simulink model "PMSM_vector_control_single"  (R2019a)
settings: Solver=ode4  StartTime=0.0  StopTime=Tfinal  FixedStep=Ts  RelTol=1e-3  EnableMultiTasking=on
values from neighbouring files (symbols this model uses):
  Cdc = 150e-6    (= 0.00015)    [PMSM_modular_vector_control_sim_parameters.m]    (also in PMSM_vector_control_single_parameters.m)
  IdPIDmax = Vdcm/5    (= 20)    [PMSM_modular_vector_control_sim_parameters.m]    (also in PMSM_vector_control_single_parameters.m)
  IdPIDmin = -Vdcm/5    (= -20)    [PMSM_modular_vector_control_sim_parameters.m]    (also in PMSM_vector_control_single_parameters.m)
  Idref = 0    [PMSM_vector_control_single_parameters.m]
  Inertia = 1e-2    (= 0.01)    [PMSM_modular_vector_control_sim_parameters.m]    (also in PMSM_vector_control_single_parameters.m)
  IqPIDmax = Vdcm-10    (= 90)    [PMSM_modular_vector_control_sim_parameters.m]    (also in PMSM_vector_control_single_parameters.m)
  IqPIDmin = -(Vdcm-10)    (= -90)    [PMSM_modular_vector_control_sim_parameters.m]    (also in PMSM_vector_control_single_parameters.m)
  IrefOverTref = MotorSpeedRad/(EfRated*3)    (= 0.261799387799)    [PMSM_modular_vector_control_sim_parameters.m]    (also in PMSM_vector_control_single_parameters.m)
  LoadTorque1 = 2    [PMSM_modular_vector_control_sim_parameters.m]    (also in PMSM_vector_control_single_parameters.m = 5)
  LoadTorque2 = 2    [PMSM_modular_vector_control_sim_parameters.m]    (also in PMSM_vector_control_single_parameters.m = 5)
  LoadTorqueStepTime = 3    [PMSM_modular_vector_control_sim_parameters.m]    (also in PMSM_vector_control_single_parameters.m)
  phase = [0 0 0 0]    [PMSM_modular_vector_control_sim_parameters.m]    (also in PMSM_vector_control_single_parameters.m)
  PolePairs = 10    [PMSM_modular_vector_control_sim_parameters.m]    (also in PMSM_vector_control_single_parameters.m)
  Rin = 1e-3    (= 0.001)    [PMSM_modular_vector_control_sim_parameters.m]    (also in PMSM_vector_control_single_parameters.m)
  Rs = 321e-3    (= 0.321)    [PMSM_modular_vector_control_sim_parameters.m]    (also in PMSM_vector_control_single_parameters.m)
  SpeedPIDmax = 20    [PMSM_modular_vector_control_sim_parameters.m]    (also in PMSM_vector_control_single_parameters.m)
  SpeedPIDmin = -20    [PMSM_modular_vector_control_sim_parameters.m]    (also in PMSM_vector_control_single_parameters.m)
  SpeedRef1 = 200    [PMSM_modular_vector_control_sim_parameters.m]    (also in PMSM_vector_control_single_parameters.m)
  SpeedRef2 = 100    [PMSM_modular_vector_control_sim_parameters.m]    (also in PMSM_vector_control_single_parameters.m)
  SpeedRefStepTime = 6    [PMSM_modular_vector_control_sim_parameters.m]    (also in PMSM_vector_control_single_parameters.m)
  Ts = 1000e-9    (= 1e-06)    [PMSM_modular_vector_control_sim_parameters.m]    (also in PMSM_vector_control_single_parameters.m)
  Vin = Vdc + Rin*(Pout/Vdc)    (= 200.01)    [PMSM_modular_vector_control_sim_parameters.m]    (also in PMSM_vector_control_single_parameters.m = 100.02)
  ViscousFriction = 1e-3    (= 0.001)    [PMSM_modular_vector_control_sim_parameters.m]    (also in PMSM_vector_control_single_parameters.m)
undefined symbols (not defined in the file or in its folder): Lload, Rload
libraries: powerlib x20, simulink x4, powerlib_meascontrol x3
settings Model: Creator=ugurm  LastModifiedBy=hakan
settings DataIOCC: LimitDataPoints=on  SaveFormat=Array  ReturnWorkspaceOutputs=off
settings OptimizationCC: LifeSpan=inf
settings DebuggingCC: UnderspecifiedInitializationDetection=Classic  MergeDetectMultiDrivingBlocksExec=none  SolverPrmCheckMsg=warning  StateNameClashWarn=warning  SFUnexpectedBacktrackingDiag=warning  SFNoUnconditionalDefaultTransitionDiag=warning  ArithmeticOperatorsInVariantConditions=warning
settings HardwareCC: ProdBitPerPointer=32  ProdBitPerSizeT=32  ProdBitPerPtrDiffT=32  ProdLargestAtomicFloat=None  ProdIntDivRoundTo=Undefined  ProdEndianess=Unspecified  ProdWordSize=32  ProdHWDeviceType=32-bit Generic
settings ModelReferenceCC: PropagateSignalLabelsOutOfModel=off
settings SFSimCC: SimUseLocalCustomCode=off
settings RTWCC: RTWUseLocalCustomCode=off
settings CodeAppCC: StateflowObjectComments=on
settings GRTTargetCC: TargetLangStandard=C89/C90 (ANSI)  GeneratePreprocessorConditionals=Disable all
settings ConfigComp: CovMetricSettings=dw  CovHtmlReporting=on  CovSaveCumulativeToWorkspaceVar=on  CovSaveSingleToWorkspaceVar=on  CovExternalEMLEnable=off
settings SimscapeCC: SimscapeNormalizeSystem=off

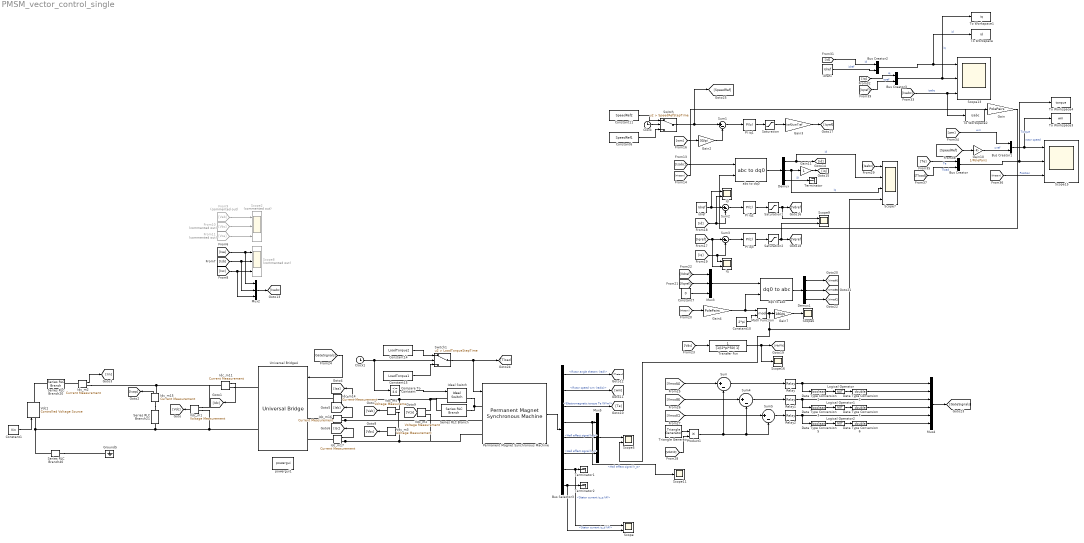
== system PMSM_vector_control_single ==
  Bus Creator{,1..3} (4 alike) : BusCreator  Inputs=2
  Bus Selector3 : BusSelector  OutputSignals=Rotor angle thetam (rad),Rotor speed wm (rad/s),Electromagnetic torque Te (N*m),Hall effect signal h_a,Hall effect signal h_b,Hall effect signal h_c,Stator current is_q (A),Stator current is_d (A)
  Clock : Clock
  Clock1 : Clock
  Compare To Constant : simulink/Logic and Bit Operations/Compare To Constant  relop=<=  const=3.0  OutDataTypeStr=boolean
  Constant1 : Constant  Value=Vin
  Constant10 : Constant  Value=2*pi
  Constant11 : Constant  Value=SpeedRef2
  Constant14 : Constant  Value=LoadTorque2
  Constant15 : Constant  Value=LoadTorque1
  Constant6 : Constant  Value=SpeedRef1
  Constant7 : Constant  Value=0
  Data Type Conversion1 : DataTypeConversion  OutDataTypeStr=boolean
  Data Type Conversion2 : DataTypeConversion  OutDataTypeStr=double
  Data Type Conversion3 : DataTypeConversion  OutDataTypeStr=boolean
  Data Type Conversion4 : DataTypeConversion  OutDataTypeStr=double
  Data Type Conversion5 : DataTypeConversion  OutDataTypeStr=boolean
  Data Type Conversion6 : DataTypeConversion  OutDataTypeStr=double
  Demux : Demux  Outputs=3
  Demux1 : Demux  Outputs=3
  From10 : From  Commented=on  GotoTag=Vbc
  From11 : From  Commented=on  GotoTag=Vca
  From9 : From  Commented=on  GotoTag=Vab
  Gain : Gain  Gain=PolePairs
  Gain10 : Gain  Gain=1/PolePairs
  Gain11 : Gain
  Gain2 : Gain  Gain=30/pi
  Gain3 : Gain  Gain=IrefOverTref
  Gain4 : Gain  Gain=PolePairs
  Gain7 : Gain  Gain=180/pi
  Ground5 : powerlib/Elements/Ground  LConnTagsString=a
      settings: SourceProductName=Simscape Electrical
  Id : Scope  NumInputPorts=2
  Idc_m{2,11,14..17} (6 alike) : powerlib/Measurements/Current Measurement  PhasorSimulation=off  OutputType=Complex  PSBequivalent=0
      settings: SourceProductName=Simscape Electrical
  Ideal Switch : powerlib/Power Electronics/Ideal Switch  Ron=0.001  Lon=0  IC=0  Rs=1e5  Cs=inf  Measurements=on
      settings: SourceProductName=Simscape Electrical
  Iq : Scope  NumInputPorts=2
  Logical Operator : Logic  Operator=NOT  AllPortsSameDT=off  OutDataTypeStr=boolean
  Logical Operator1 : Logic  Operator=NOT  AllPortsSameDT=off  OutDataTypeStr=boolean
  Logical Operator2 : Logic  Operator=NOT  AllPortsSameDT=off  OutDataTypeStr=boolean
  Math Function : Math  Operator=mod  SaturateOnIntegerOverflow=on
  Mux2 : Mux  Inputs=3
  Mux3 : Mux  Inputs=3
  Mux4 : Mux  Inputs=6
  Mux5 : Mux  Inputs=3
  PI iq1 : simulink/Continuous/PID Controller  Controller=PI  Form=Parallel  TimeDomain=Discrete-time  SampleTime=-1  IntegratorMethod=Forward Euler  FilterMethod=Forward Euler  ControllerParametersSource=internal  P=0.1  I=1  D=0  UseFilter=on  N=100  TunerSelectOption=Transfer Function Based (PID Tuner App)  InitialConditionSource=internal  InitialConditionForIntegrator=0  InitialConditionForFilter=0  DifferentiatorICPrevScaledInput=0  ExternalReset=none  TrackingMode=off  Kt=1  LimitOutput=off  UpperSaturationLimit=inf  LowerSaturationLimit=-inf  LinearizeAsGain=on  AntiWindupMode=none  Kb=1  POutMin=[]  POutMax=[]  IOutMin=[]  IOutMax=[]  DOutMin=[]  DOutMax=[]  NOutMin=[]  NOutMax=[]  SumOutMin=[]  SumOutMax=[]  SaturationOutMin=[]  SaturationOutMax=[]  PParamMin=[]  PParamMax=[]  IParamMin=[]  IParamMax=[]  DParamMin=[]  DParamMax=[]  NParamMin=[]  NParamMax=[]  KbParamMin=[]  KbParamMax=[]  KtParamMin=[]  KtParamMax=[]  KbOutMin=[]  KbOutMax=[]  KtOutMin=[]  KtOutMax=[]  IntegratorOutMin=[]  IntegratorOutMax=[]  FilterOutMin=[]  FilterOutMax=[]  SumI1OutMin=[]  SumI1OutMax=[]  SumI2OutMin=[]  SumI2OutMax=[]  SumI3OutMin=[]  SumI3OutMax=[]  SumI4OutMin=[]  SumI4OutMax=[]  SumDOutMin=[]  SumDOutMax=[]  DifferentiatorOutMin=[]  DifferentiatorOutMax=[]  FilterDiffOutCoefMin=[]  FilterDiffOutCoefMax=[]  ReciprocalOutMin=[]  ReciprocalOutMax=[]  SumDenOutMin=[]  SumDenOutMax=[]  SumNumOutMin=[]  SumNumOutMax=[]  DivideOutMin=[]  DivideOutMax=[]  IntegratorContinuousStateAttributes=''  IntegratorStateMustResolveToSignalObject=off  IntegratorRTWStateStorageClass=Auto  FilterContinuousStateAttributes=''  FilterStateMustResolveToSignalObject=off  FilterRTWStateStorageClass=Auto  ParallelPVariant=InternalParameters  IdealPVariant=Disabled  IVariant=InternalParameters  DVariant=Disabled  IntegratorVariant=Discrete  SatVariant=Disabled  AWVariant=Passthrough  PCopyVariant=Disabled  TRVariant=Disabled  FdbkBlocksVariant=Forward  IdealPFdbkVariant=Disabled  SatFdbkVariant=Disabled  DerivativeFilterVariant=Disabled  NVariant=Disabled  NCopyVariant=Disabled_SignalSpec  FilterICVariant=Disabled  IntegratorICVariant=InternalICs  ExternalResetVariant=Disabled  TRSumVariant=Passthrough  SumFdbkVariant=Disabled  SumVariant=Sum_PI
  PI iq2 : simulink/Continuous/PID Controller  Controller=PI  Form=Parallel  TimeDomain=Discrete-time  SampleTime=-1  IntegratorMethod=Forward Euler  FilterMethod=Forward Euler  ControllerParametersSource=internal  P=100  I=100  D=0  UseFilter=on  N=100  TunerSelectOption=Transfer Function Based (PID Tuner App)  InitialConditionSource=internal  InitialConditionForIntegrator=0  InitialConditionForFilter=0  DifferentiatorICPrevScaledInput=0  ExternalReset=none  TrackingMode=off  Kt=1  LimitOutput=off  UpperSaturationLimit=inf  LowerSaturationLimit=-inf  LinearizeAsGain=on  AntiWindupMode=none  Kb=1  POutMin=[]  POutMax=[]  IOutMin=[]  IOutMax=[]  DOutMin=[]  DOutMax=[]  NOutMin=[]  NOutMax=[]  SumOutMin=[]  SumOutMax=[]  SaturationOutMin=[]  SaturationOutMax=[]  PParamMin=[]  PParamMax=[]  IParamMin=[]  IParamMax=[]  DParamMin=[]  DParamMax=[]  NParamMin=[]  NParamMax=[]  KbParamMin=[]  KbParamMax=[]  KtParamMin=[]  KtParamMax=[]  KbOutMin=[]  KbOutMax=[]  KtOutMin=[]  KtOutMax=[]  IntegratorOutMin=[]  IntegratorOutMax=[]  FilterOutMin=[]  FilterOutMax=[]  SumI1OutMin=[]  SumI1OutMax=[]  SumI2OutMin=[]  SumI2OutMax=[]  SumI3OutMin=[]  SumI3OutMax=[]  SumI4OutMin=[]  SumI4OutMax=[]  SumDOutMin=[]  SumDOutMax=[]  DifferentiatorOutMin=[]  DifferentiatorOutMax=[]  FilterDiffOutCoefMin=[]  FilterDiffOutCoefMax=[]  ReciprocalOutMin=[]  ReciprocalOutMax=[]  SumDenOutMin=[]  SumDenOutMax=[]  SumNumOutMin=[]  SumNumOutMax=[]  DivideOutMin=[]  DivideOutMax=[]  IntegratorContinuousStateAttributes=''  IntegratorStateMustResolveToSignalObject=off  IntegratorRTWStateStorageClass=Auto  FilterContinuousStateAttributes=''  FilterStateMustResolveToSignalObject=off  FilterRTWStateStorageClass=Auto  ParallelPVariant=InternalParameters  IdealPVariant=Disabled  IVariant=InternalParameters  DVariant=Disabled  IntegratorVariant=Discrete  SatVariant=Disabled  AWVariant=Passthrough  PCopyVariant=Disabled  TRVariant=Disabled  FdbkBlocksVariant=Forward  IdealPFdbkVariant=Disabled  SatFdbkVariant=Disabled  DerivativeFilterVariant=Disabled  NVariant=Disabled  NCopyVariant=Disabled_SignalSpec  FilterICVariant=Disabled  IntegratorICVariant=InternalICs  ExternalResetVariant=Disabled  TRSumVariant=Passthrough  SumFdbkVariant=Disabled  SumVariant=Sum_PI
  PI iq3 : simulink/Continuous/PID Controller  Controller=PI  Form=Parallel  TimeDomain=Discrete-time  SampleTime=-1  IntegratorMethod=Forward Euler  FilterMethod=Forward Euler  ControllerParametersSource=internal  P=100  I=100  D=0  UseFilter=on  N=100  TunerSelectOption=Transfer Function Based (PID Tuner App)  InitialConditionSource=internal  InitialConditionForIntegrator=0  InitialConditionForFilter=0  DifferentiatorICPrevScaledInput=0  ExternalReset=none  TrackingMode=off  Kt=1  LimitOutput=off  UpperSaturationLimit=inf  LowerSaturationLimit=-inf  LinearizeAsGain=on  AntiWindupMode=none  Kb=1  POutMin=[]  POutMax=[]  IOutMin=[]  IOutMax=[]  DOutMin=[]  DOutMax=[]  NOutMin=[]  NOutMax=[]  SumOutMin=[]  SumOutMax=[]  SaturationOutMin=[]  SaturationOutMax=[]  PParamMin=[]  PParamMax=[]  IParamMin=[]  IParamMax=[]  DParamMin=[]  DParamMax=[]  NParamMin=[]  NParamMax=[]  KbParamMin=[]  KbParamMax=[]  KtParamMin=[]  KtParamMax=[]  KbOutMin=[]  KbOutMax=[]  KtOutMin=[]  KtOutMax=[]  IntegratorOutMin=[]  IntegratorOutMax=[]  FilterOutMin=[]  FilterOutMax=[]  SumI1OutMin=[]  SumI1OutMax=[]  SumI2OutMin=[]  SumI2OutMax=[]  SumI3OutMin=[]  SumI3OutMax=[]  SumI4OutMin=[]  SumI4OutMax=[]  SumDOutMin=[]  SumDOutMax=[]  DifferentiatorOutMin=[]  DifferentiatorOutMax=[]  FilterDiffOutCoefMin=[]  FilterDiffOutCoefMax=[]  ReciprocalOutMin=[]  ReciprocalOutMax=[]  SumDenOutMin=[]  SumDenOutMax=[]  SumNumOutMin=[]  SumNumOutMax=[]  DivideOutMin=[]  DivideOutMax=[]  IntegratorContinuousStateAttributes=''  IntegratorStateMustResolveToSignalObject=off  IntegratorRTWStateStorageClass=Auto  FilterContinuousStateAttributes=''  FilterStateMustResolveToSignalObject=off  FilterRTWStateStorageClass=Auto  ParallelPVariant=InternalParameters  IdealPVariant=Disabled  IVariant=InternalParameters  DVariant=Disabled  IntegratorVariant=Discrete  SatVariant=Disabled  AWVariant=Passthrough  PCopyVariant=Disabled  TRVariant=Disabled  FdbkBlocksVariant=Forward  IdealPFdbkVariant=Disabled  SatFdbkVariant=Disabled  DerivativeFilterVariant=Disabled  NVariant=Disabled  NCopyVariant=Disabled_SignalSpec  FilterICVariant=Disabled  IntegratorICVariant=InternalICs  ExternalResetVariant=Disabled  TRSumVariant=Passthrough  SumFdbkVariant=Disabled  SumVariant=Sum_PI
  Permanent Magnet Synchronous Machine : powerlib/Machines/Permanent Magnet Synchronous Machine  NbPhases=3  FluxDistribution=Sinusoidal  RotorType=Round  MechanicalLoad=Torque Tm  PresetModel=No  ShowDetailedParameters=on  MeasurementBus=off  Resistance=Rs  Inductance=8.5e-3  dqInductances=[3.1e-3,3.6e-3]  La=Ls  MachineConstant=Voltage Constant (V_peak L-L / krpm)  Flux=0.18006  VoltageCst=VoltageConstant  TorqueCst=2.7009  Flat=120  Mechanical=[Inertia ViscousFriction PolePairs 0]  PolePairs=4  InitialConditions=[0,0, 0,0]  InitialConditions5ph=[0 0 0 0 0 0]  TsPowergui=0  TsBlock=-1  RefAngle=90 degrees behind phase A axis (modified Park)
  Product1 : Product
  Relay : Relay
  Relay1 : Relay
  Relay2 : Relay
  Saturation : Saturate  UpperLimit=SpeedPIDmax  LowerLimit=SpeedPIDmin
  Saturation1 : Saturate  UpperLimit=IdPIDmax  LowerLimit=IdPIDmin
  Saturation2 : Saturate  UpperLimit=IqPIDmax  LowerLimit=IqPIDmin
  Scope : Scope  NumInputPorts=2
  Scope11 : Scope
  Scope13 : Scope  NumInputPorts=3
  Scope15 : Scope  NumInputPorts=3
  Scope16 : Scope
  Scope2 : Scope  Commented=on  NumInputPorts=3
  Scope5 : Scope  NumInputPorts=2
  Scope6 : Scope
  Scope7 : Scope  NumInputPorts=4
  Scope8 : Scope  Commented=on  NumInputPorts=3
  Scope9 : Scope  NumInputPorts=2
  Series RLC Branch : powerlib/Elements/Series RLC Branch  LConnTagsString=__new0  RConnTagsString=__new0  BranchType=R  Resistance=5000  Inductance=1e-3  SetiL0=off  InitialCurrent=0  Capacitance=1e-6  Setx0=off  InitialVoltage=0  Measurements=None
      settings: SourceProductName=Simscape Electrical
  Series RLC Branch20 : powerlib/Elements/Series RLC Branch  LConnTagsString=__new0  RConnTagsString=__new0  BranchType=R  Resistance=Rin  Inductance=1e-3  SetiL0=off  InitialCurrent=0  Capacitance=1e-6  Setx0=off  InitialVoltage=0  Measurements=None
      settings: SourceProductName=Simscape Electrical
  Series RLC Branch21 : powerlib/Elements/Series RLC Branch  LConnTagsString=__new0  RConnTagsString=__new0  BranchType=C  Resistance=Rload  Inductance=Lload  SetiL0=off  InitialCurrent=0  Capacitance=Cdc  Setx0=off  InitialVoltage=0  Measurements=None
      settings: SourceProductName=Simscape Electrical
  Series RLC Branch40 : powerlib/Elements/Series RLC Branch  LConnTagsString=__new0  RConnTagsString=__new0  BranchType=R  Resistance=1e12  Inductance=Lload  SetiL0=off  InitialCurrent=0  Capacitance=1e-6  Setx0=off  InitialVoltage=0  Measurements=None
      settings: SourceProductName=Simscape Electrical
  Sum{,1..5} (6 alike) : Sum  Inputs=|+-
  Switch : Switch  Criteria=u2 > Threshold  Threshold=SpeedRefStepTime
  Switch1 : Switch  Criteria=u2 > Threshold  Threshold=LoadTorqueStepTime
  Terminator : Terminator
  Terminator1 : Terminator
  Terminator2 : Terminator
  To Workspace : ToWorkspace  VariableName=id  SaveFormat=Timeseries  SampleTime=-1
  To Workspace1 : ToWorkspace  VariableName=iq  SaveFormat=Timeseries  SampleTime=-1
  To Workspace2 : ToWorkspace  VariableName=isabc  SaveFormat=Timeseries  SampleTime=-1
  To Workspace3 : ToWorkspace  VariableName=wm  SaveFormat=Timeseries  SampleTime=-1
  To Workspace4 : ToWorkspace  VariableName=torque  SaveFormat=Timeseries  SampleTime=-1
  Transfer Fcn : TransferFcn  Denominator=[1/(2*pi*50) 1]
  Triangle Generator : powerlib_meascontrol/Pulse & Signal Generators/Triangle Generator  Freq=fsw  Phase=phase(1)  Ts=Ts
      settings: SourceProductName=Simscape Electrical
  Universal Bridge4 : powerlib/Power Electronics/Universal Bridge  Arms=3  SnubberResistance=1e5  SnubberCapacitance=inf  Device=IGBT / Diodes  Ron=1e-6  Lon=0  ForwardVoltages="[  0  0  ]"  ForwardVoltage=0  GTOparameters=[ 10e-6 , 20e-6 ]  IGBTparameters=[0,0]  Measurements=None  Measurements_2=None  converterType=Rectifier
      settings: SourceProductName=Simscape Electrical
  Vdc1 : powerlib/Electrical Sources/Controlled Voltage Source  Initialize=off  Source_Type=DC  Amplitude=200  Phase=0  Frequency=0  Measurements=None
      settings: SourceProductName=Simscape Electrical
  Vdc_m{1..3,5} (4 alike) : powerlib/Measurements/Voltage Measurement  PhasorSimulation=off  OutputType=Complex  PSBequivalent=0
      settings: SourceProductName=Simscape Electrical
  abc to dq0 : powerlib_meascontrol/Transformations/abc to dq0  Alignment=90 degrees behind phase A axis
      settings: SourceProductName=Simscape Electrical
  dq0 to abc : powerlib_meascontrol/Transformations/dq0 to abc  Alignment=90 degrees behind phase A axis
      settings: SourceProductName=Simscape Electrical
  idref : Constant  Value=Idref
  idref1 : Constant  Value=Idref
  powergui1 : powerlib/powergui  Priority=1  SimulationMode=Discrete  SampleTime=Ts  frequency=60  Iterations=50  frequencyindice=0  Pbase=100e6  ErrMax=1e-4  UnitsV=kV  UnitsW=MW  buscounter=0  FunctionMessages=off  echomessages=off  EnableUseOfTLC=off  CurrentSourceSwitches=off  DisableSnubberDevices=off  DisableRonSwitches=off  DisableVfSwitches=off  DisplayEquations=off  AutomaticDiscreteSolvers=off  SolverType=Tustin  Interpol=off  ExternalGateDelay=off  methode=off  Ts=0  x0status=blocks  SPID=off  SwTol=0  HookPort=off  NonlinearTolerance=0  nMaxIteration=15  ContinueOnMaxIteration=off  RestoreLinks=warning  ResistiveCurrentMeasurement=off  Frange=[0:2:500]  Ylog=off  Xlog=on  ShowGrid=off  save=off  variable=ZData  structure=Icap  ZoomFFT=off  StartTime=0.04  cycles=5  DisplayStyle=3  fundamental=150  FreqAxis=off  MaxFrequency=1000  frequencyindicesteady=1  RmsSteady=1  display=off
      settings: SourceProductName=Simscape Electrical
  wires:
  Idc_m14/1 -> [Isa]
  Constant1/1 -> Vdc1/1
  Idc_m15/1 -> [Icap]
  Idc_m16/1 -> [Isb]
  Idc_m17/1 -> [Isc]
  Idc_m11/1 -> [Idc]
  Vdc_m1/1 -> [Vdc]
  Idc_m2/1 -> [Iin]
  Vdc_m5/1 -> [Vab]
  Vdc_m3/1 -> [Vbc]
  Vdc_m2/1 -> [Vca]
  [Isa] -> Mux2/1, Scope8/1
  [Isb] -> Mux2/2, Scope8/2
  [Isc] -> Mux2/3, Scope8/3
  From9/1 -> Scope2/1
  From10/1 -> Scope2/2
  From11/1 -> Scope2/3
  Permanent Magnet Synchronous Machine/1 -> Bus Selector3/1
  Bus Selector3/3 -> [Te]  "<Electromagnetic torque Te (N*m)>"
  Bus Selector3/2 -> [wm]  "<Rotor speed wm (rad/s)>"
  Bus Selector3/1 -> [Thetam]  "<Rotor angle thetam (rad)>"
  Mux2/1 -> [Isabc]
  [Isabc] -> abc to dq0/1
  Gain/1 -> abc to dq0/2
  [Thetam] -> Gain/1
  abc to dq0/1 -> Demux/1
  Demux/1 -> [id], Scope7/2  "id"
  Demux/2 -> Gain11/1, Scope7/3  "iq"
  Demux/3 -> Terminator/1  "i0"
  [wm] -> Gain2/1
  Gain2/1 -> Sum1/2
  Switch/1 -> [SpeedRef], Sum1/1
  Sum1/1 -> PI iq1/1
  PI iq1/1 -> Saturation/1
  Saturation/1 -> Gain3/1
  Gain3/1 -> [Iqref]
  [id] -> Id/2, Sum2/2
  Sum2/1 -> PI iq2/1
  PI iq2/1 -> Saturation1/1
  idref/1 -> Id/1, Sum2/1
  [iq] -> Iq/1, Sum3/2
  Sum3/1 -> PI iq3/1
  PI iq3/1 -> Saturation2/1
  [Iqref] -> Iq/2, Sum3/1
  Saturation2/1 -> [Vqref], Scope9/2
  [Thetam] -> Gain4/1
  Gain4/1 -> Math Function/1, dq0 to abc/2
  Constant7/1 -> Mux3/3
  Mux3/1 -> dq0 to abc/1
  [Vdc] -> Transfer Fcn/1
  Transfer Fcn/1 -> Scope16/1, [VdcFilt]
  dq0 to abc/1 -> Demux1/1
  Sum/1 -> Relay/1
  Sum4/1 -> Relay1/1
  Sum5/1 -> Relay2/1
  Data Type Conversion1/1 -> Logical Operator/1
  Logical Operator/1 -> Data Type Conversion2/1
  Data Type Conversion2/1 -> Mux4/2
  Data Type Conversion3/1 -> Logical Operator1/1
  Relay1/1 -> Data Type Conversion3/1, Mux4/3
  Logical Operator1/1 -> Data Type Conversion4/1
  Data Type Conversion4/1 -> Mux4/4
  Data Type Conversion5/1 -> Logical Operator2/1
  Relay2/1 -> Data Type Conversion5/1, Mux4/5
  Logical Operator2/1 -> Data Type Conversion6/1
  Data Type Conversion6/1 -> Mux4/6
  Relay/1 -> Mux4/1, Data Type Conversion1/1
  [VmodC] -> Sum5/1
  Triangle Generator/1 -> Product1/1
  [VdcFilt] -> Product1/2
  Demux1/1 -> [VmodA]
  Demux1/2 -> [VmodB]
  Demux1/3 -> [VmodC]
  Mux4/1 -> [GateSignals]
  Switch1/1 -> [Tload], Permanent Magnet Synchronous Machine/1
  [GateSignals] -> Universal Bridge4/1
  Product1/1 -> Sum/2, Sum4/2, Sum5/2
  Bus Selector3/6 -> Mux5/3  "<Hall effect signal h_c>"
  Bus Selector3/5 -> Mux5/2  "<Hall effect signal h_b>"
  Bus Selector3/4 -> Scope11/1, Mux5/1  "<Hall effect signal h_a>"
  Mux5/1 -> Scope5/1
  Constant10/1 -> Math Function/2
  Math Function/1 -> Scope7/4, Scope5/2, Gain7/1
  Gain7/1 -> Scope6/1
  [Isabc] -> Scope7/1
  Gain11/1 -> [iq]
  Bus Selector3/7 -> Scope/1, Terminator1/1  "<Stator current is_q (A)>"
  Bus Selector3/8 -> Scope/2, Terminator2/1  "<Stator current is_d (A)>"
  Saturation1/1 -> [Vdref], Scope9/1
  [Vqref] -> Mux3/2
  [Vdref] -> Mux3/1
  Clock/1 -> Switch/2
  Constant11/1 -> Switch/1
  Constant6/1 -> Switch/3
  Clock1/1 -> Compare To Constant/1, Switch1/2
  Constant14/1 -> Switch1/1
  Constant15/1 -> Switch1/3
  [VmodA] -> Sum/1
  [VmodB] -> Sum4/1
  Bus Creator3/1 -> To Workspace1/1, Scope13/2  "iq"
  [Isabc] -> To Workspace2/1, Scope13/3  "isabc"
  [Thetam] -> Scope15/3  "Position"
  Compare To Constant/1 -> Ideal Switch/1
  [Te] -> Bus Creator/1  "Te"
  [Tload] -> Bus Creator/2  "Tload"
  Bus Creator/1 -> To Workspace4/1, Scope15/2  "Torque"
  Bus Creator1/1 -> To Workspace3/1, Scope15/1  "rotor speed"
  [wm] -> Bus Creator1/1  "wm"
  [SpeedRef] -> Gain10/1
  idref1/1 -> Bus Creator2/2  "idref"
  [id] -> Bus Creator2/1  "id"
  Bus Creator2/1 -> To Workspace/1, Scope13/1  "id"
  [iq] -> Bus Creator3/1  "iq"
  [Iqref] -> Bus Creator3/2  "iqref"
  Gain10/1 -> Bus Creator1/2  "wref"
  connections:
  Vdc_m5/LConn1 -- Series RLC Branch/LConn1 -- Ideal Switch/LConn1 -- Vdc_m2/LConn2 -- Idc_m14/RConn1
  Series RLC Branch40/RConn1 -- Ground5/LConn1
  Idc_m14/LConn1 -- Universal Bridge4/LConn1
  Idc_m15/LConn1 -- Series RLC Branch21/LConn1
  Vdc1/RConn1 -- Series RLC Branch20/LConn1
  Idc_m16/LConn1 -- Universal Bridge4/LConn2
  Idc_m17/LConn1 -- Universal Bridge4/LConn3
  Idc_m17/RConn1 -- Permanent Magnet Synchronous Machine/LConn3 -- Vdc_m2/LConn1 -- Vdc_m3/LConn2
  Idc_m16/RConn1 -- Permanent Magnet Synchronous Machine/LConn2 -- Vdc_m3/LConn1 -- Vdc_m5/LConn2
  Idc_m15/RConn1 -- Idc_m11/LConn1 -- Vdc_m1/LConn1 -- Idc_m2/RConn1
  Idc_m11/RConn1 -- Universal Bridge4/RConn1
  Vdc_m1/LConn2 -- Universal Bridge4/RConn2 -- Series RLC Branch21/RConn1 -- Vdc1/LConn1 -- Series RLC Branch40/LConn1
  Idc_m2/LConn1 -- Series RLC Branch20/RConn1
  Ideal Switch/RConn1 -- Series RLC Branch/RConn1 -- Permanent Magnet Synchronous Machine/LConn1
